simulink library "cdma2000_lib"  (Simulink 6.0)
settings: Solver=ode45  SolverMode=SingleTasking  StartTime=0.0  StopTime=10.0  RelTol=1e-3
values from neighbouring files (symbols this model uses):
  numTapsChEst = str2num(Vals{idxNumTapsChEst})    [wcdma_initmaskphlayer.m]    (also in wcdma_initmaskspreadandmod.m; wcdma_loadinitphlayer.m = 21; wcdma_loadinitspreadandmod.m = 21)
  overSampling = str2num(Vals{idxOverSampling})    [wcdma_initmaskphlayer.m]    (also in wcdma_initmaskspreadandmod.m; wcdma_loadinitphlayer.m = 8; wcdma_loadinitspreadandmod.m = 8)
undefined symbols (not defined in the file or in its folder): decPattern, gateRate, j, longCodeScrOff, magnitude, numPuncturedSymbols, numSymbPCGroup, overSamp, PCGroupInit, plcm_37, powerControlOff, qof_sign, scrBitRepetition, symbolTime, walshLength
libraries: dspsigops x30, dspsrcs4 x29, commutil2 x14, cdma2000_lib x13, commseqgen2 x10, dspbuff3 x9, dspsigattribs x7, dspindex x5, commsequence2 x4, commchan2 x3, simulink x3, dspmtrx3 x2
(part 2 of 2)

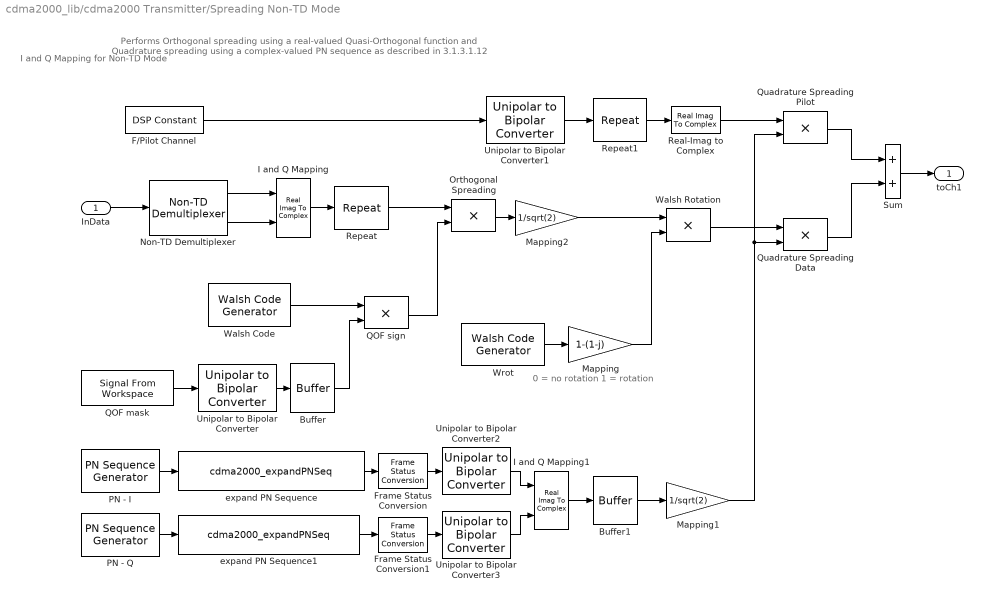
== system cdma2000_lib/cdma2000 Transmitter/Spreading Non-TD Mode ==
  note: I and Q Mapping for Non-TD Mode
  note: 0 = no rotation
      | 1 = rotation
  note: Performs Orthogonal spreading using a real-valued Quasi-Orthogonal function
      | and Quadrature spreading using a complex-valued PN sequence as described in 3.1.3.1.12
  InData : Inport  LatchInput=off
  Buffer : dspbuff3/Buffer  N=walshLength  V=0  ic=0
      settings: AttributesFormatString=\n
  Buffer1 : dspbuff3/Buffer  N=walshLength  V=0  ic=0
      settings: AttributesFormatString=\n
  F/Pilot Channel : dspsrcs4/DSP Constant  Value=0  SampleMode=Discrete  discreteOutput=Frame-based  continuousOutput=Sample-based  sampTime=1  framePeriod=64/1.2288e6  dataType=Inherit from 'Constant value'  isSigned=on  wordLen=16  udDataType=sfix(16)  fracBitsMode=Best precision  numFracBits=15  InterpretAs1D=-inf  Ts=-inf  FramebasedOutput=-inf
  Frame Status Conversion : dspsigattribs/Frame Status Conversion  growRefPort=off  outframe=Frame-based
  Frame Status Conversion1 : dspsigattribs/Frame Status Conversion  growRefPort=off  outframe=Frame-based
  I and Q Mapping : RealImagToComplex
  I and Q Mapping1 : RealImagToComplex
  Mapping : Gain  Gain=1-(1-j)  SaturateOnIntegerOverflow=on
  Mapping1 : Gain  Gain=1/sqrt(2)  SaturateOnIntegerOverflow=on
  Mapping2 : Gain  Gain=1/sqrt(2)  SaturateOnIntegerOverflow=on
  Non-TD Demultiplexer : cdma2000_lib/cdma2000 Transmitter/Non-TD Demultiplexer
  Orthogonal Spreading : Product  SaturateOnIntegerOverflow=on
  PN - I : commseqgen2/PN Sequence Generator  poly=[15 13 9 8 7 5 0]  ini_sta=[1 zeros(1,14)]  shift=14+pnOffset*64  Ts=2/(75*(2^15-1))  frameBased=on  sampPerFrame=2^15-1  reset=off
  PN - Q : commseqgen2/PN Sequence Generator  poly=[15 12 11 10 6 5 4 3 0]  ini_sta=[1 zeros(1,14)]  shift=14+pnOffset*64  Ts=2/(75*(2^15-1))  frameBased=on  sampPerFrame=2^15-1  reset=off
  QOF mask : dspsrcs4/Signal From Workspace  X=qof_sign(qof_idx,:)  Ts=1/1.2288e6  nsamps=256  OutputAfterFinalValue=Cyclic repetition
  QOF sign : Product  SaturateOnIntegerOverflow=on
  Quadrature Spreading Data : Product  SaturateOnIntegerOverflow=on
  Quadrature Spreading Pilot : Product  SaturateOnIntegerOverflow=on
  Real-Imag to Complex : RealImagToComplex  Input=Real
  Repeat : dspsigops/Repeat  N=walshLength  ic=0  mode=Maintain input frame rate
  Repeat1 : dspsigops/Repeat  N=64  ic=0  mode=Maintain input frame rate
  Sum : Sum  SaturateOnIntegerOverflow=on
  Unipolar to Bipolar Converter{,1..3} (4 alike) : commutil2/Unipolar to Bipolar Converter  M=2  polarity=Negative
  Walsh Rotation : Product  SaturateOnIntegerOverflow=on
  Walsh Code : commseqgen2/Walsh Code Generator  length=walshLength  index=trChCode  ts=1/1.2288e6  frameBased=on  sampPerFrame=walshLength
  Wrot : commseqgen2/Walsh Code Generator  length=256  index=walshRotIdx(qof_idx)  ts=1/1.2288e6  frameBased=on  sampPerFrame=walshLength
  expand PN Sequence : S-Function  FunctionName=cdma2000_expandPNSeq  SFunctionModules=cdma2000_expandPNSeq_wrapper  WizardData=DataTag1  mask(S-Function Builder){}
      mask init:
      | val = [[.9  0.75 0.75 1 1 .9 .9 1]',[1 1 0.75 0.75 .9 .9 1 .9]'];try , sys = get_param(gcb,'SfunBuilderFcnName');if isempty(sys), sys = get_param(gcb,'FunctionName'); end,catch, sys = get_param(gcb,'FunctionName'); end
      settings: CopyFcn=set_param(gcb,'LinkStatus','none')  OpenFcn=sfunctionwizard(gcbh)
      mask Display: plot(val(:,1),val(:,2)),disp(sys)port_label('input',1,'inPN')port_label('output',1,'outPN')
  expand PN Sequence1 : S-Function  FunctionName=cdma2000_expandPNSeq  SFunctionModules=cdma2000_expandPNSeq_wrapper  WizardData=DataTag2  mask(S-Function Builder){}
      mask init: same as cdma2000_lib/cdma2000 Transmitter/Spreading Non-TD Mode/expand PN Sequence
      settings: CopyFcn=set_param(gcb,'LinkStatus','none')  OpenFcn=sfunctionwizard(gcbh)
      mask Display: plot(val(:,1),val(:,2)),disp(sys)port_label('input',1,'inPN')port_label('output',1,'outPN')
  toCh1 : Outport
  wires:
  I and Q Mapping/1 -> Repeat/1
  Walsh Code/1 -> QOF sign/1
  QOF sign/1 -> Orthogonal Spreading/2
  Repeat/1 -> Orthogonal Spreading/1
  QOF mask/1 -> Unipolar to Bipolar Converter/1
  Buffer/1 -> QOF sign/2
  Orthogonal Spreading/1 -> Mapping2/1
  Wrot/1 -> Mapping/1
  Unipolar to Bipolar Converter/1 -> Buffer/1
  Mapping/1 -> Walsh Rotation/2
  Walsh Rotation/1 -> Quadrature Spreading Data/1
  I and Q Mapping1/1 -> Buffer1/1
  PN - I/1 -> expand PN Sequence/1
  Frame Status Conversion/1 -> Unipolar to Bipolar Converter2/1
  Frame Status Conversion1/1 -> Unipolar to Bipolar Converter3/1
  Buffer1/1 -> Mapping1/1
  Non-TD Demultiplexer/1 -> I and Q Mapping/1
  Non-TD Demultiplexer/2 -> I and Q Mapping/2
  InData/1 -> Non-TD Demultiplexer/1
  expand PN Sequence/1 -> Frame Status Conversion/1
  Quadrature Spreading Pilot/1 -> Sum/1
  Quadrature Spreading Data/1 -> Sum/2
  Sum/1 -> toCh1/1
  F/Pilot Channel/1 -> Unipolar to Bipolar Converter1/1
  Unipolar to Bipolar Converter1/1 -> Repeat1/1
  Repeat1/1 -> Real-Imag to Complex/1
  Real-Imag to Complex/1 -> Quadrature Spreading Pilot/1
  Mapping1/1 -> Quadrature Spreading Data/2, Quadrature Spreading Pilot/2
  Mapping2/1 -> Walsh Rotation/1
  Unipolar to Bipolar Converter2/1 -> I and Q Mapping1/1
  Unipolar to Bipolar Converter3/1 -> I and Q Mapping1/2
  PN - Q/1 -> expand PN Sequence1/1
  expand PN Sequence1/1 -> Frame Status Conversion1/1

== system cdma2000_lib/cdma2000 Transmitter/Tx Channel Structure ==
  note: Performs Frame Quality Indicator and tail bits attachment, convolutional encoding with rate 1/4 constraint length 9,
      | repeatition and puncturing as described in Figure 3.1.3.1.1.1-15
  note: Tx Channel Structure for
      | Forward Fundamental Channel - Radio Configuration 3
  Ch Bits : Inport  LatchInput=off
  Add FQI : commcrc2/General CRC Generator  genPoly=[6 5 2 1 0]  iniStates=[1]  numChecksums=1
  Block Interleaver : commblkintrlv2/General Block Interleaver  elements=interTable
  Convolutional Encoder : commcnvcod2/Convolutional Encoder  trellis=poly2trellis(9, [765 671 513 473])  reset=On each frame
  Encoder Tail Bits : dspsigops/Zero Pad  padSigAt=End  zpadAlong=Columns  padNumOutRowsSpecMethod=User-specified  numOutRows=16 + 6 + 8  padNumOutColsSpecMethod=User-specified  numOutCols=1  trunc_flag=None
  Puncture : commsequence2/Puncture  punctureVector=[1;1;1;1;0]
  Repeat : dspsigops/Repeat  N=8  ic=0  mode=Maintain input frame rate
  Mod Symbols : Outport
  wires:
  Puncture/1 -> Block Interleaver/1
  Repeat/1 -> Puncture/1
  Convolutional Encoder/1 -> Repeat/1
  Encoder Tail Bits/1 -> Convolutional Encoder/1
  Add FQI/1 -> Encoder Tail Bits/1
  Ch Bits/1 -> Add FQI/1
  Block Interleaver/1 -> Mod Symbols/1

== system cdma2000_lib/cdma2000 Receiver/Long Code DeScrambling Power Control Extracting/Hard Decisions ==
  In1 : Inport  LatchInput=off
  Bipolar to Unipolar Converter : commutil2/Bipolar to Unipolar Converter  M=2  polarity=Negative
  Sign : Signum
  Out1 : Outport
  wires:
  In1/1 -> Sign/1
  Bipolar to Unipolar Converter/1 -> Out1/1
  Sign/1 -> Bipolar to Unipolar Converter/1

== system cdma2000_lib/cdma2000 Receiver/Long Code DeScrambling Power Control Extracting/Power Control Bit Position Extractor ==
  note: Compute Power Control Bit Position for Power Control subchannel as described in TIA/EIA/IS-2000.2.A 3.1.3.1.10
  note: Power Control Bit Position
      | Extractor
  Decimated Bits : Inport  LatchInput=off
  Enable : EnablePort
  Bit to Integer Converter : commutil2/Bit to Integer Converter  nbits=length(decPattern)
  Buffer : dspbuff3/Buffer  N=numSymbPCGroup  V=0  ic=0
      settings: AttributesFormatString=\n
  Decimator1 : dspindex/Multiport Selector  rowsOrCols=Rows  idxCellArray={decPattern}  idxErrMode=Clip Index
      settings: AttributesFormatString=\n
  Starting Symbol Position : Gain  Gain=2*scrBitRepetition  SaturateOnIntegerOverflow=on
  Bits : Outport
  wires:
  Bit to Integer Converter/1 -> Starting Symbol Position/1
  Buffer/1 -> Decimator1/1
  Decimator1/1 -> Bit to Integer Converter/1
  Decimated Bits/1 -> Buffer/1
  Starting Symbol Position/1 -> Bits/1

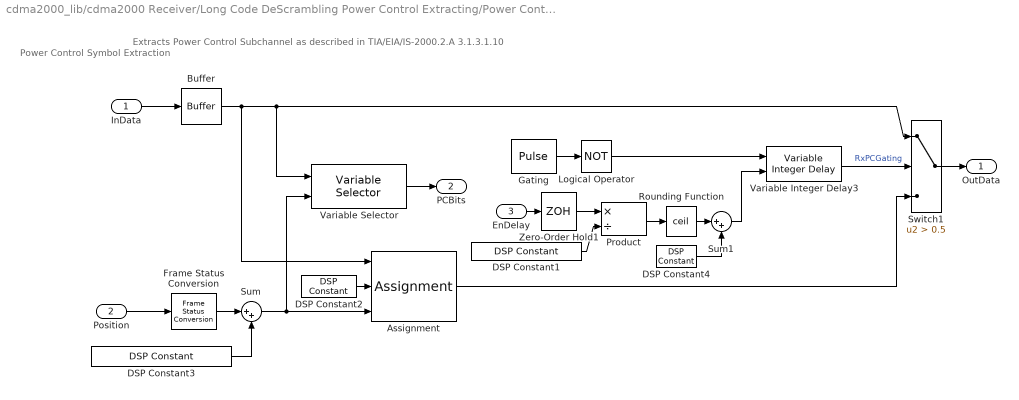
== system cdma2000_lib/cdma2000 Receiver/Long Code DeScrambling Power Control Extracting/Power Control Symbol Extraction ==
  note: Power Control Symbol Extraction
  note: Extracts Power Control Subchannel as described in TIA/EIA/IS-2000.2.A 3.1.3.1.10
  InData : Inport  LatchInput=off
  Position : Inport  Port=2  LatchInput=off
  EnDelay : Inport  Port=3  LatchInput=off
  Assignment : Assignment  ElementSrc=External
  Buffer : dspbuff3/Buffer  N=numSamp/16  V=0  ic=0
  DSP Constant1 : dspsrcs4/DSP Constant  Value=numSamp/(2*16)  SampleMode=Discrete  discreteOutput=Sample-based  continuousOutput=Sample-based  sampTime=20e-3/16  framePeriod=20e-3/16  dataType=Inherit from 'Constant value'  wordLen=16  udDataType=sfix(16)  fracBitsMode=Best precision  numFracBits=15  InterpretAs1D=off  Ts=20e-3/16  FramebasedOutput=off
  DSP Constant2 : dspsrcs4/DSP Constant  Value=0  SampleMode=Discrete  discreteOutput=Sample-based  continuousOutput=Sample-based  sampTime=1.25e-3  framePeriod=1.25e-3  dataType=Inherit from 'Constant value'  wordLen=16  udDataType=sfix(16)  fracBitsMode=Best precision  numFracBits=15  InterpretAs1D=off  Ts=1.25e-3  FramebasedOutput=off
  DSP Constant3 : dspsrcs4/DSP Constant  Value=[1:numPuncturedSymbols]  SampleMode=Discrete  discreteOutput=Sample-based  continuousOutput=Sample-based  sampTime=1.25e-3  framePeriod=1.25e-3  dataType=Inherit from 'Constant value'  wordLen=16  udDataType=sfix(16)  fracBitsMode=Best precision  numFracBits=15  InterpretAs1D=off  Ts=1.25e-3  FramebasedOutput=off
  DSP Constant4 : dspsrcs4/DSP Constant  Value=1  SampleMode=Discrete  discreteOutput=Sample-based  continuousOutput=Sample-based  sampTime=1.25e-3  framePeriod=1.25e-3  dataType=Inherit from 'Constant value'  wordLen=16  udDataType=sfix(16)  fracBitsMode=Best precision  numFracBits=15  InterpretAs1D=off  Ts=1.25e-3  FramebasedOutput=off
  Frame Status Conversion : dspsigattribs/Frame Status Conversion  growRefPort=off  outframe=Sample-based
  Gating : DiscretePulseGenerator  Amplitude=powerControlOff  Period=1/gateRate  PhaseDelay=PCGroupInit  SampleTime=20e-3/16
  Logical Operator : Logic  Operator=NOT  AllPortsSameDT=off
  Product : Product  Inputs=*/  SaturateOnIntegerOverflow=on
  Rounding Function : Rounding  Operator=ceil
  Sum : Sum  Inputs=|++  SaturateOnIntegerOverflow=on
  Sum1 : Sum  Inputs=|++  SaturateOnIntegerOverflow=on
  Switch1 : Switch  Criteria=u2 > Threshold  Threshold=0.5  SaturateOnIntegerOverflow=on
  Variable Integer Delay3 : dspsigops/Variable Integer Delay  dmax=numSamp+10  ic=1
  Variable Selector : dspindex/Variable Selector  rowsOrCols=Rows  IdxMode=Variable  Elements=[1 3]  ZerOneIdxMode=One-based  errmode=Clip Index
  Zero-Order Hold1 : ZeroOrderHold  SampleTime=20e-3/16
  OutData : Outport
  PCBits : Outport  Port=2
  wires:
  DSP Constant4/1 -> Sum1/2
  Sum1/1 -> Variable Integer Delay3/2
  Rounding Function/1 -> Sum1/1
  Zero-Order Hold1/1 -> Product/1
  Product/1 -> Rounding Function/1
  DSP Constant1/1 -> Product/2
  EnDelay/1 -> Zero-Order Hold1/1
  Variable Integer Delay3/1 -> Switch1/2  "RxPCGating"
  Logical Operator/1 -> Variable Integer Delay3/1
  Gating/1 -> Logical Operator/1
  Position/1 -> Frame Status Conversion/1
  Variable Selector/1 -> PCBits/1
  Assignment/1 -> Switch1/3
  Frame Status Conversion/1 -> Sum/1
  DSP Constant2/1 -> Assignment/2
  Sum/1 -> Variable Selector/2, Assignment/3
  DSP Constant3/1 -> Sum/2
  Buffer/1 -> Switch1/1, Variable Selector/1, Assignment/1
  InData/1 -> Buffer/1
  Switch1/1 -> OutData/1

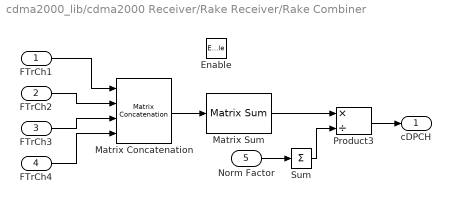
== system cdma2000_lib/cdma2000 Receiver/Rake Receiver/Rake Combiner ==
  FTrCh1 : Inport  LatchInput=off
  FTrCh2 : Inport  Port=2  LatchInput=off
  FTrCh3 : Inport  Port=3  LatchInput=off
  FTrCh4 : Inport  Port=4  LatchInput=off
  Norm Factor : Inport  Port=5  LatchInput=off
  Enable : EnablePort
  Matrix Concatenation : simulink/Math Operations/Matrix Concatenation  numInports=4  catMethod=Horizontal
  Matrix Sum : dspmtrx3/Matrix Sum  Dim=Rows  roundingMode=Floor  overflowMode=off
  Product3 : Product  Inputs=*/  SaturateOnIntegerOverflow=on  InputSameDT=on
  Sum : Sum  Inputs=+  SaturateOnIntegerOverflow=on  InputSameDT=on
  cDPCH : Outport
  wires:
  Product3/1 -> cDPCH/1
  Norm Factor/1 -> Sum/1
  Sum/1 -> Product3/2
  Matrix Concatenation/1 -> Matrix Sum/1
  FTrCh1/1 -> Matrix Concatenation/1
  FTrCh2/1 -> Matrix Concatenation/2
  FTrCh3/1 -> Matrix Concatenation/3
  FTrCh4/1 -> Matrix Concatenation/4
  Matrix Sum/1 -> Product3/1

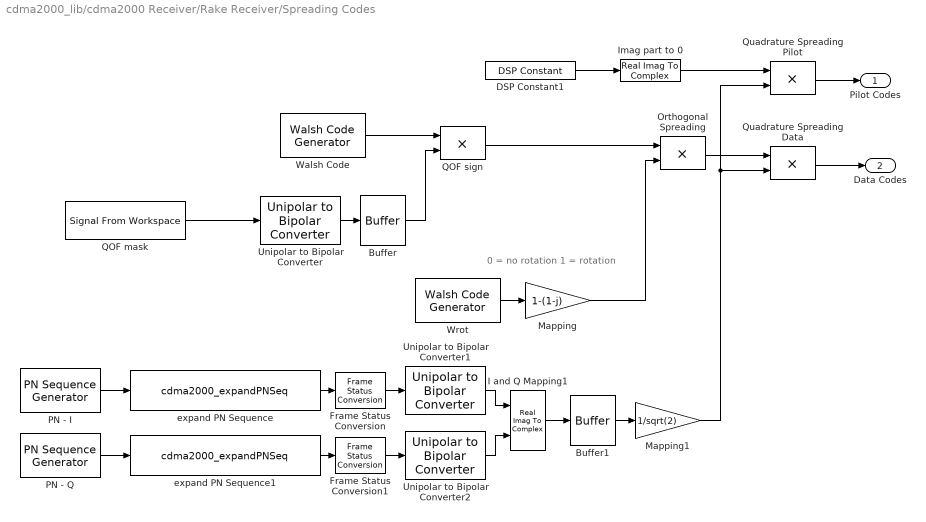
== system cdma2000_lib/cdma2000 Receiver/Rake Receiver/Spreading Codes ==
  note: 0 = no rotation
      | 1 = rotation
  Buffer : dspbuff3/Buffer  N=walshLength  V=0  ic=0
      settings: AttributesFormatString=\n
  Buffer1 : dspbuff3/Buffer  N=walshLength  V=0  ic=0
      settings: AttributesFormatString=\n
  DSP Constant1 : dspsrcs4/DSP Constant  Value=1  SampleMode=Discrete  discreteOutput=Frame-based  continuousOutput=Sample-based  sampTime=64/1.2288e6  framePeriod=64/1.2288e6  dataType=Inherit from 'Constant value'  wordLen=16  udDataType=sfix(16)  fracBitsMode=Best precision  numFracBits=15  InterpretAs1D=off  Ts=64/1.2288e6  FramebasedOutput=on
  Frame Status Conversion : dspsigattribs/Frame Status Conversion  growRefPort=off  outframe=Frame-based
  Frame Status Conversion1 : dspsigattribs/Frame Status Conversion  growRefPort=off  outframe=Frame-based
  I and Q Mapping1 : RealImagToComplex
  Imag part to 0 : RealImagToComplex  Input=Real
  Mapping : Gain  Gain=1-(1-j)  SaturateOnIntegerOverflow=on
  Mapping1 : Gain  Gain=1/sqrt(2)  SaturateOnIntegerOverflow=on
  Orthogonal Spreading : Product  SaturateOnIntegerOverflow=on
  PN - I : commseqgen2/PN Sequence Generator  poly=[15 13 9 8 7 5 0]  ini_sta=[1 zeros(1,14)]  shift=14+pnOffset*64  Ts=2/(75*(2^15-1))  frameBased=on  sampPerFrame=2^15-1  reset=off
  PN - Q : commseqgen2/PN Sequence Generator  poly=[15 12 11 10 6 5 4 3 0]  ini_sta=[1 zeros(1,14)]  shift=14+pnOffset*64  Ts=2/(75*(2^15-1))  frameBased=on  sampPerFrame=2^15-1  reset=off
  QOF mask : dspsrcs4/Signal From Workspace  X=qof_sign(qof_idx,:)  Ts=1/1.2288e6  nsamps=256  OutputAfterFinalValue=Cyclic repetition
  QOF sign : Product  SaturateOnIntegerOverflow=on
  Quadrature Spreading Data : Product  SaturateOnIntegerOverflow=on
  Quadrature Spreading Pilot : Product  SaturateOnIntegerOverflow=on
  Unipolar to Bipolar Converter : commutil2/Unipolar to Bipolar Converter  M=2  polarity=Negative
  Unipolar to Bipolar Converter1 : commutil2/Unipolar to Bipolar Converter  M=2  polarity=Negative
  Unipolar to Bipolar Converter2 : commutil2/Unipolar to Bipolar Converter  M=2  polarity=Negative
  Walsh Code : commseqgen2/Walsh Code Generator  length=walshLength  index=trChCode  ts=1/1.2288e6  frameBased=on  sampPerFrame=walshLength
  Wrot : commseqgen2/Walsh Code Generator  length=256  index=walshRotIdx(qof_idx)  ts=1/1.2288e6  frameBased=on  sampPerFrame=walshLength
  expand PN Sequence : S-Function  FunctionName=cdma2000_expandPNSeq  SFunctionModules=cdma2000_expandPNSeq_wrapper  WizardData=DataTag0  mask(S-Function Builder){}
      mask init: same as cdma2000_lib/cdma2000 Transmitter/Spreading Non-TD Mode/expand PN Sequence
      settings: CopyFcn=set_param(gcb,'LinkStatus','none')  OpenFcn=sfunctionwizard(gcbh)
      mask Display: plot(val(:,1),val(:,2)),disp(sys)port_label('input',1,'inPN')port_label('output',1,'outPN')
  expand PN Sequence1 : S-Function  FunctionName=cdma2000_expandPNSeq  SFunctionModules=cdma2000_expandPNSeq_wrapper  mask(S-Function Builder){}
      mask init: same as cdma2000_lib/cdma2000 Transmitter/Spreading Non-TD Mode/expand PN Sequence
      settings: CopyFcn=set_param(gcb,'LinkStatus','none')  OpenFcn=sfunctionwizard(gcbh)
      mask Display: plot(val(:,1),val(:,2)),disp(sys)port_label('input',1,'inPN')port_label('output',1,'outPN')
  Pilot Codes : Outport
  Data Codes : Outport  Port=2
  wires:
  Mapping1/1 -> Quadrature Spreading Data/2, Quadrature Spreading Pilot/2
  Unipolar to Bipolar Converter2/1 -> I and Q Mapping1/2
  Unipolar to Bipolar Converter1/1 -> I and Q Mapping1/1
  Walsh Code/1 -> QOF sign/1
  QOF mask/1 -> Unipolar to Bipolar Converter/1
  Buffer/1 -> QOF sign/2
  Unipolar to Bipolar Converter/1 -> Buffer/1
  QOF sign/1 -> Orthogonal Spreading/1
  Wrot/1 -> Mapping/1
  Mapping/1 -> Orthogonal Spreading/2
  I and Q Mapping1/1 -> Buffer1/1
  PN - I/1 -> expand PN Sequence/1
  PN - Q/1 -> expand PN Sequence1/1
  Frame Status Conversion/1 -> Unipolar to Bipolar Converter1/1
  Frame Status Conversion1/1 -> Unipolar to Bipolar Converter2/1
  expand PN Sequence/1 -> Frame Status Conversion/1
  expand PN Sequence1/1 -> Frame Status Conversion1/1
  Orthogonal Spreading/1 -> Quadrature Spreading Data/1
  Buffer1/1 -> Mapping1/1
  Quadrature Spreading Data/1 -> Data Codes/1
  DSP Constant1/1 -> Imag part to 0/1
  Quadrature Spreading Pilot/1 -> Pilot Codes/1
  Imag part to 0/1 -> Quadrature Spreading Pilot/1

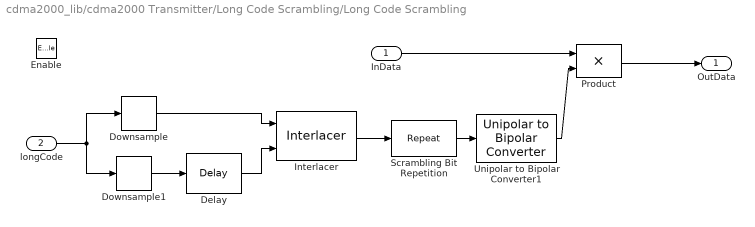
== system cdma2000_lib/cdma2000 Transmitter/Long Code Scrambling/Long Code Scrambling ==
  InData : Inport  LatchInput=off
  longCode : Inport  Port=2  LatchInput=off
  Enable : EnablePort
  Delay : dspsigops/Delay  dly_unit=Samples  delay=1  ic_detail=off  dif_ic_for_ch=off  dif_ic_for_dly=off  ic=0  reset_popup=None
  Downsample : dspsigops/Downsample  N=64  phase=0  ic=0  smode=Allow multirate  fmode=Maintain input frame rate
  Downsample1 : dspsigops/Downsample  N=64  phase=63  ic=0  smode=Allow multirate  fmode=Maintain input frame rate
  Interlacer : commsequence2/Interlacer
  Product : Product  SaturateOnIntegerOverflow=on
  Scrambling Bit Repetition : dspsigops/Repeat  N=scrBitRepetition  ic=0  mode=Maintain input frame rate
  Unipolar to Bipolar Converter1 : commutil2/Unipolar to Bipolar Converter  M=2  polarity=Negative
  OutData : Outport
  wires:
  Product/1 -> OutData/1
  InData/1 -> Product/1
  longCode/1 -> Downsample/1, Downsample1/1
  Delay/1 -> Interlacer/2
  Downsample1/1 -> Delay/1
  Downsample/1 -> Interlacer/1
  Interlacer/1 -> Scrambling Bit Repetition/1
  Unipolar to Bipolar Converter1/1 -> Product/2
  Scrambling Bit Repetition/1 -> Unipolar to Bipolar Converter1/1
